simulink model "lqi12_discreto"  (R2025b)
settings: Solver=VariableStepAuto  StartTime=0.0  StopTime=30  RelTol=1e-3
values from neighbouring files (symbols this model uses):
  Cm = [1 0 0 0 0 0 0 0 0 0 1 0 ... (108 elements, 9x12)]    [parametros_LQI.mat]
  D = [0 0 0 0 0 0 0 0 0 0 0 0 ... (36 elements, 9x4)]    [parametros_LQI.mat]
  K = [8.61388977208e-09 -3.23938755891e-11 27.1624608635 1.22408347835e-11 5.15548702544e-09 -26.9052309444 4.91703547324e-11 2.27757364143e-13 56.1282376315 -9.6103215742e-14 8.73666069887e-14 -5.56559839576e-15 ... (64 elements, 4x16)]    [parametros_LQI.mat]
undefined symbols (not defined in the file or in its folder): C, Discrete, L, sys, Time
libraries: ctrlSharedLib x1, simulink x1, uavutilslib x1
settings Model: Creator=rel  LastModifiedBy=labro

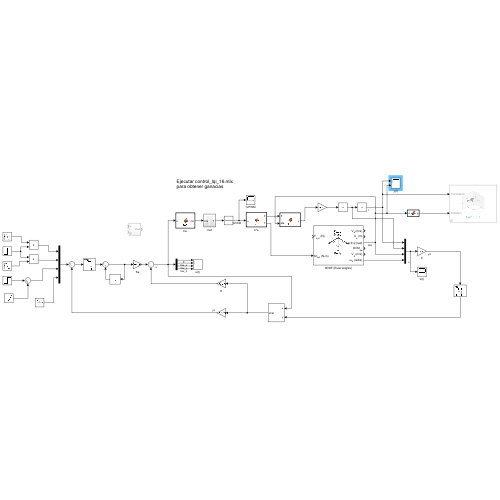
[thumbnail: Simulink's stored preview of the top-level diagram]
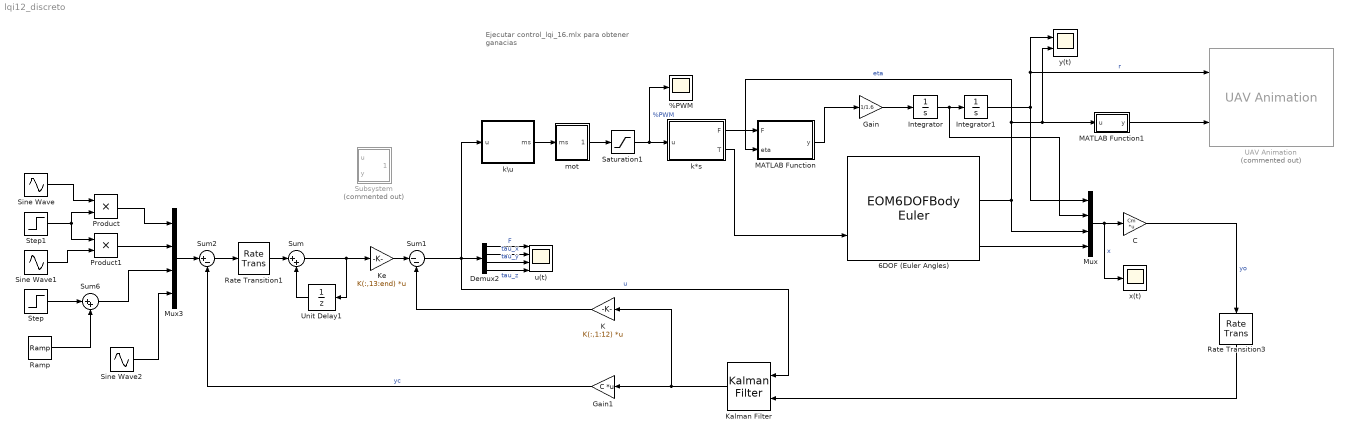
== system lqi12_discreto ==
  note: Ejecutar control_lqi_16.mlx
      | para obtener ganacias
  %PWM : Scope
      settings: ActiveDisplayYMinimum=-0.1061075392828715  ActiveDisplayYMaximum=0.95496785354584379  DataLoggingVariableName=ScopeData4
  6DOF (Euler Angles) : EOM6DOFBodyEuler  mass_0=1.6  inertia=diag([0.021915027 0.022124548 0.042349865])
  C : Gain  Gain=Cm  Multiplication=Matrix(K*u) (u vector)
  Demux2 : Demux
  Gain : Gain  Gain=1/1.6
  Gain1 : Gain  Gain=C  Multiplication=Matrix(K*u) (u vector)
  Integrator : Integrator
  Integrator1 : Integrator
  K : Gain  Gain=K(:,1:12)  Multiplication=Matrix(K*u) (u vector)
  Kalman Filter : ctrlSharedLib/Kalman Filter  TimeDomain=Discrete-Time  UseCurrentEstimator=on  ModelSource=LTI State-Space Variable  ModelSourceVariable=ss(sys.A, sys.B, Cm, D, 1/100)  A=0.95  B=1  C=1  D=0  NumberOfStates=1  NumberOfInputs=1  NumberOfOutputs=1  InitialEstimateSource=Dialog  X0=0  P0=10  UseK=off  UseGH=off  NumberOfProcessNoiseInputs=1  G=1  TimeInvariantG=on  H=0  TimeInvariantH=on  Q=0.05  TimeInvariantQ=on  R=1  TimeInvariantR=on  N=0  TimeInvariantN=on  AddInputPort=on  AddEnablePort=off  OutputEstimatedY=off  OutputP=off  Ts=-1
  Ke : Gain  Gain=K(:,13:end)  Multiplication=Matrix(K*u) (u vector)
  MATLAB Function : MATLAB Function  TreatAsAtomicUnit=on
  MATLAB Function1 : MATLAB Function  TreatAsAtomicUnit=on
  Mux : Mux
  Mux3 : Mux
  Product : Product
  Product1 : Product
  Ramp : simulink/Sources/Ramp  slope=1/60  start=2  InitialOutput=0
  Rate Transition1 : RateTransition  OutPortSampleTime=1/100
  Rate Transition3 : RateTransition
  Saturation1 : Saturate  UpperLimit=1  LowerLimit=0
  Sine Wave : Sin  Amplitude=0.5  Bias=0.2  Frequency=3  SampleTime=0
  Sine Wave1 : Sin  Amplitude=0.5  Bias=0.2  Phase=pi/2  SampleTime=0
  Sine Wave2 : Sin  Amplitude=deg2rad(30)  SampleTime=0
  Step : Step  SampleTime=0
  Step1 : Step  Time=3  SampleTime=0
  Subsystem : Subsystem  Commented=on
  Sum : Sum  Inputs=|++
  Sum1 : Sum  Inputs=|--
  Sum2 : Sum  Inputs=|+-
  Sum6 : Sum  Inputs=|++
  UAV Animation : uavutilslib/UAV Animation  Commented=on  NumUAV=1  DynamicUAVConfig=off  UAVType=Multirotor  UAVSize=1  UAVColor=[1 0 0]  UAVTrajectoryAlpha=1  InertialZDirection=Up  RotationFormat=Euler ZYX  DrawMarkers=off  SampleTime=1/100
  Unit Delay1 : UnitDelay  SampleTime=1/100  HasFrameUpgradeWarning=on
  k*s : MATLAB Function  TreatAsAtomicUnit=on
  k\u : MATLAB Function  TreatAsAtomicUnit=on
  mot : Subsystem
  u(t) : Scope  NumInputPorts=4
      settings: ActiveDisplayYMinimum=-4.6710350826190856  ActiveDisplayYMaximum=7.730689684176892
  x(t) : Scope
      settings: ActiveDisplayYMinimum=-1.6070132129490062  ActiveDisplayYMaximum=1.6076444329729518  DataLoggingVariableName=ScopeData3
  y(t) : Scope  NumInputPorts=2
      settings: ActiveDisplayYMinimum=-0.87074066068786848  ActiveDisplayYMaximum=1.7057012443274961
  wires:
  K/1 -> Sum1/2
  Sum/1 -> Ke/1, Unit Delay1/1
  6DOF (Euler Angles)/3 -> y(t)/2, MATLAB Function1/1(u), MATLAB Function/2(eta), Mux/3  "eta"
  mot/1(Out1) -> Saturation1/1
  k\u/1(ms) -> mot/1(ms)
  Saturation1/1 -> %PWM/1, k*s/1(u)  "%PWM"
  k*s/2(T) -> 6DOF (Euler Angles)/2
  k*s/1(F) -> MATLAB Function/1(F)
  Integrator/1 -> Mux/2, Integrator1/1
  6DOF (Euler Angles)/6 -> Mux/4
  Mux/1 -> x(t)/1, C/1  "x"
  Unit Delay1/1 -> Sum/2
  Sum2/1 -> Rate Transition1/1
  Ke/1 -> Sum1/1
  Sine Wave2/1 -> Mux3/4
  Demux2/1 -> u(t)/1  "F"
  Demux2/2 -> u(t)/2  "tau_x"
  Demux2/3 -> u(t)/3  "tau_y"
  Demux2/4 -> u(t)/4  "tau_z"
  Gain/1 -> Integrator/1
  MATLAB Function/1(y) -> Gain/1
  Integrator1/1 -> Mux/1, y(t)/1, UAV Animation/1  "r"
  C/1 -> Rate Transition3/1  "yo"
  Sum1/1 -> k\u/1(u), Kalman Filter/1, Demux2/1  "u"
  Product1/1 -> Mux3/2
  Product/1 -> Mux3/1
  Sine Wave1/1 -> Product1/2
  Sine Wave/1 -> Product/1
  Step1/1 -> Product1/1, Product/2
  Step/1 -> Sum6/1
  Ramp/1 -> Sum6/2
  Sum6/1 -> Mux3/3
  MATLAB Function1/1(y) -> UAV Animation/2
  Rate Transition3/1 -> Kalman Filter/2
  Kalman Filter/1 -> Gain1/1, K/1
  Mux3/1 -> Sum2/1
  Rate Transition1/1 -> Sum/1
  Gain1/1 -> Sum2/2  "yc"

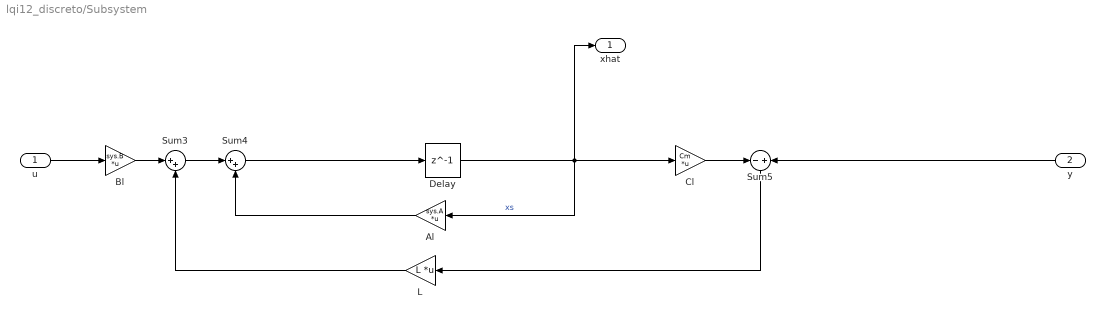
== system lqi12_discreto/Subsystem ==
  u : Inport
  y : Inport  Port=2
  Al : Gain  Gain=sys.A  Multiplication=Matrix(K*u) (u vector)
  Bl : Gain  Gain=sys.B  Multiplication=Matrix(K*u) (u vector)
  Cl : Gain  Gain=Cm  Multiplication=Matrix(K*u)
  Delay : Delay  DelayLength=1
  L : Gain  Gain=L  Multiplication=Matrix(K*u) (u vector)
  Sum3 : Sum  Inputs=|++
  Sum4 : Sum  Inputs=|++
  Sum5 : Sum  Inputs=-|+
  xhat : Outport
  wires:
  Sum3/1 -> Sum4/1
  Sum5/1 -> L/1
  Delay/1 -> xhat/1, Al/1, Cl/1  "xs"
  L/1 -> Sum3/2
  Bl/1 -> Sum3/1
  Cl/1 -> Sum5/1
  Sum4/1 -> Delay/1
  Al/1 -> Sum4/2
  u/1 -> Bl/1
  y/1 -> Sum5/2

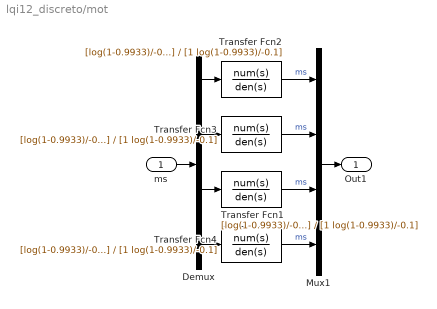
== system lqi12_discreto/mot ==
  ms : Inport
  Demux : Demux
  Mux1 : Mux
  Transfer Fcn{1..4} (4 alike) : TransferFcn  Numerator=[log(1-0.9933)/-0.1]  Denominator=[1 log(1-0.9933)/-0.1]
  Out1 : Outport
  wires:
  Transfer Fcn3/1 -> Mux1/2  "ms"
  Transfer Fcn1/1 -> Mux1/3  "ms"
  Demux/3 -> Transfer Fcn1/1
  Transfer Fcn4/1 -> Mux1/4  "ms"
  Demux/4 -> Transfer Fcn4/1
  Mux1/1 -> Out1/1
  Transfer Fcn2/1 -> Mux1/1  "ms"
  Demux/2 -> Transfer Fcn3/1
  Demux/1 -> Transfer Fcn2/1
  ms/1 -> Demux/1

== matlab function lqi12_discreto/k\u ==
  data: u input; ms output
function ms = fcn(u)
% L = 0.0080;
% kF = 0.1600*9.81;
% kM = 0.0086;
L = 0.268554;
kF = 7.965;
kM = 0.2;
A = [kF kF kF kF; -L*kF -L*kF L*kF L*kF; L*kF -L*kF -L*kF L*kF; -kM kM -kM kM];
ms = A\[u(1)+1*9.81*1.6; u(2:end)];

== matlab function lqi12_discreto/MATLAB Function ==
  data: F input; y output; eta input
function y = fcn(F, eta)
phi = eta(1);
theta = eta(2);
psi = eta(3);
y = [0;0;-1.6*9.81] + [sin(theta)*cos(psi) + sin(phi)*cos(theta)*sin(psi); ...
                    sin(theta)*sin(psi) - sin(phi)*cos(theta)*cos(psi); ...
                    cos(phi)*cos(theta)]*F;

== matlab function lqi12_discreto/k*s ==
  data: u input; F output; T output
function [F, T] = fcn(u)
% L = 0.0080;
% kF = 0.1600*9.81;
% kM = 0.0086;
L = 0.268554;
kF = 7.965;
kM = 0.2;
A = [kF kF kF kF; -L*kF -L*kF L*kF L*kF; L*kF -L*kF -L*kF L*kF; -kM kM -kM kM];
y = A*u;
F = y(1);
T = y(2:end);

== matlab function lqi12_discreto/MATLAB Function1 ==
  data: u input; y output
function y = fcn(u)
y = flip(u);
